simulink model "Servoclef"  (R2019b)
settings: Solver=VariableStepAuto  StartTime=0.0  StopTime=0.5  RelTol=1e-3
settings Model: Creator=jeanz  LastModifiedBy=jeanz

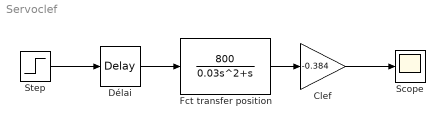
== system Servoclef ==
  Clef : Gain  Gain=-0.384
  Délai : TransportDelay  DelayTime=0.01
  Fct transfer position : TransferFcn  Numerator=[800]  Denominator=[0.03 1 0]
  Scope : Scope
  Step : Step  Time=0.03  SampleTime=0
  wires:
  Délai/1 -> Fct transfer position/1
  Fct transfer position/1 -> Clef/1
  Clef/1 -> Scope/1
  Step/1 -> Délai/1
